simulink model "mech_bouncing_ball"  (Simulink 6.0)
settings: Solver=ode15s  StartTime=0.0  StopTime=20  FixedStep=.01  RelTol=1e-3
PreLoadFcn:
  | ball.radius = 0.2; ball.pengain = 1e5;
  | ball.mass = 1; ball.pendamp = 25;
values from neighbouring files (symbols this model uses):
  m = 161    [mech_transmission_data.mat]
  N = 270    [mech_transmission_data.mat]
libraries: mblibv1 x8
settings Model: Creator=jwendlan  LastModifiedBy=batserve  ExtModeAutoUpdateStatusClock=off  ProdHWDeviceType=Specified
settings DataIOCC: SignalLoggingName=sigsOut  OutputOption=SpecifiedOutputTimes  OutputTimes=[0:0.1:20]  Refine=3
settings DebuggingCC: CheckExecutionContextPreStartOutputMsg=on  CheckExecutionContextRuntimeOutputMsg=on  SolverPrmCheckMsg=none
settings HardwareCC: ProdHWDeviceType=Specified
settings CodeAppCC: MangleLength=5
settings SimMechanicsCC: VisOnUpdateDiagram=on  VisDuringSimulation=on  VisConfigFile=mech_bouncing_ball.mat

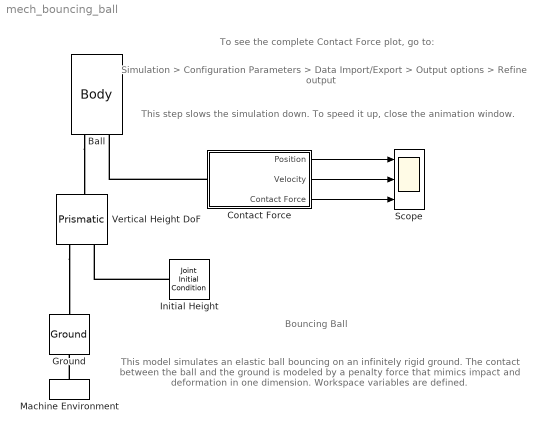
== system mech_bouncing_ball ==
  note: Bouncing Ball
  note: This model simulates an elastic ball bouncing on
      | an infinitely rigid ground. The contact between
      | the ball and the ground is modeled by a penalty force
      | that mimics impact and deformation in
      | one dimension. Workspace variables are defined.
  note: To see the complete Contact Force plot, go to:
  note: Simulation > Configuration Parameters >
      | Data Import/Export > Output options >
      | Refine output
  note: This step slows the simulation down. To speed it
      | up, close the animation window.
  Ball : mblibv1/Bodies/Body  Orientation=up  PhysicalDomain=mechanical  SubClassName=Unknown  LeftPortType=workingframe  RightPortType=workingframe  LConnTagsString=CS1|CG  DialogClass=MechanicalBodyBlock  Mass=ball.mass  MassUnits=kg  InertiaUnits=kg*m^2  Inertia=eye(3)*(2/5)*ball.mass*ball.radius^2  Shape=Cylinder  ShapeDims=[1 1]  ShapeUnits=m  ShapeUse=false  Density=1  DensityUnits=kg/m^3  DensityUse=false  CG=Left$CG$[0 0 ball.radius]$CS1$CS1$m$[0 0 0]$Euler X-Y-Z$deg$WORLD$true  WorkingFrames=Left$CS1$[0 0 0]$ADJOINING$ADJOINING$m$[0 0 0]$Euler X-Y-Z$deg$WORLD$true
  Contact Force : Subsystem
  Ground : mblibv1/Bodies/Ground  Orientation=up  Opaque=on  LeftPortType=env  RightPortType=workingframe  PhysicalDomain=Mechanical  DialogClass=GroundBlock  CoordPosition=[0 0 0]  CoordPositionUnits=m  StateVectorMgrId=-1  MachineId=[0 0]  ShowEnvPort=on
  Initial Height : mblibv1/Sensors &  Actuators/Joint Initial Condition  Orientation=left  Opaque=on  PhysicalDomain=Mechanical  DialogClass=InitialConditionBlock  InitialConditions=P1$true$5$m$rad$0$m/s$rad/s#P2$false$0$m$rad$0$m/s$rad/s#P3$false$0$m$rad$0$m/s$rad/s#R1$false$0$m$rad$0$m/s$rad/s#R2$false$0$m$rad$0$m/s$rad/s#R3$false$0$m$rad$0$m/s$rad/s#S$false$0$m$rad$0$m/s$rad/s
  Machine Environment : mblibv1/Bodies/Machine Environment  Tag=Factory ground  Orientation=up  DialogController=MECH.DialogSource  Opaque=on  PortType=env  PhysicalDomain=Mechanical  DialogTemplateClass=MECH.MachineEnvironment  SyncWhenCopied=off  Gravity=[0 0 -9.81]  GravityUnits=m/s^2  GravityAsSignal=off  Dimensionality=3D Only  AnalysisType=Forward dynamics  LinearAssemblyTolerance=1e-3  LinearAssemblyToleranceUnits=m  AngularAssemblyTolerance=1e-3  AngularAssemblyToleranceUnits=rad  ConstraintSolverType=Stabilizing  ConstraintRelTolerance=1e-4  ConstraintAbsTolerance=1e-4  UseRobustSingularityHandling=off  StatePerturbationType=Fixed  PerturbationSize=1e-5  VisualizeMachine=on
  Scope : Scope  NumInputPorts=3
      settings: TimeRange=20  YMin=0~-10~0  YMax=6~10~3000  MaxDataPoints=50000
  Vertical Height DoF : mblibv1/Joints/Prismatic  Orientation=up  PhysicalDomain=mechanical  SubClassName=Unknown  LeftPortType=blob  RightPortType=blob  LConnTagsString=__newl0|SA1  RConnTagsString=__newr0  NumSAPorts=1  CutJoint=off  MarkAsCut=off  Primitives=prismatic  PrimitiveProps=P1$WORLD$[0 0 1]$prismatic  DialogClass=JointBlock
  wires:
  Contact Force/1(Position) -> Scope/1
  Contact Force/2(Velocity) -> Scope/2
  Contact Force/3(Contact Force) -> Scope/3
  connections:
  Vertical Height DoF/LConn1 -- Ground/RConn1
  Initial Height/RConn1 -- Vertical Height DoF/LConn2
  Ball/LConn1 -- Vertical Height DoF/RConn1
  Contact Force/LConn1 -- Ball/LConn2
  Machine Environment/RConn1 -- Ground/LConn1

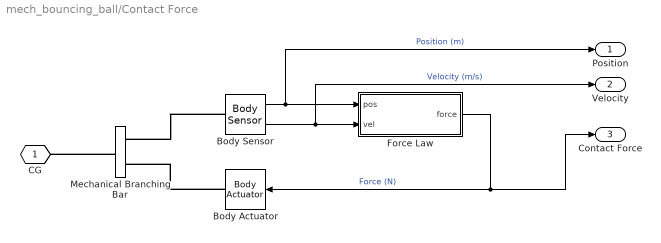
== system mech_bouncing_ball/Contact Force ==
  Body Actuator : mblibv1/Sensors &  Actuators/Body Actuator  Orientation=left  Opaque=on  PhysicalDomain=Mechanical  PortType=blob  ActuationStyle=Force  AngleUnits=deg  ArcVelocityUnits=deg/s  ArcAccelerationUnits=deg/s^2  CoordPositionUnits=m  VelocityUnits=m/s  AccelerationUnits=m/s^2  ForceUnits=N  TorqueUnits=N-m  ActiveIO=on  Width=3  DialogClass=MechanicalActuatorBlock  ReferenceFrame=Absolute (INERTIAL)  Angle=off  CoordPosition=on  Force=on  Torque=off
  Body Sensor : mblibv1/Sensors &  Actuators/Body Sensor  Opaque=on  PhysicalDomain=Mechanical  PortType=blob  Muxed=off  Pose=off  Angle=on  AngleUnits=deg  ArcVelocity=off  ArcVelocityUnits=deg/s  ArcAcceleration=off  ArcAccelerationUnits=deg/s^2  CoordPosition=on  CoordPositionUnits=m  Velocity=on  VelocityUnits=m/s  Acceleration=off  AccelerationUnits=m/s^2  Quaternion=on  QuaternionDT=off  QuaternionDDT=off  QuaternionUnits=off  OutputVector=[ 3 3 ]  ActiveIO=on  Width=6  DialogClass=MechanicalSensorBlock  ReferenceFrame=Absolute (World)
  Force Law : Subsystem
  Mechanical Branching Bar : mblibv1/Utilities/Mechanical Branching Bar  PhysicalDomain=mechanical  SubClassName=Unknown  LeftPortType=blob  RightPortType=blob  LConnTagsString=_newl0  RConnTagsString=SA0|SA1  DialogClass=MechanicalBranchingBarBlock  NumSAPorts=2
  CG : PMIOPort  Tag=PMCPort  Port=1  Side=Left
  Position : Outport
  Velocity : Outport  Port=2
  Contact Force : Outport  Port=3
  wires:
  Body Sensor/1 -> Force Law/1(pos), Position/1  "Position (m)"
  Body Sensor/2 -> Force Law/2(vel), Velocity/1  "Velocity (m/s)"
  Force Law/1(force) -> Body Actuator/1, Contact Force/1  "Force (N)"
  connections:
  Mechanical Branching Bar/LConn1 -- CG/RConn1
  Body Actuator/RConn1 -- Mechanical Branching Bar/RConn2
  Body Sensor/LConn1 -- Mechanical Branching Bar/RConn1

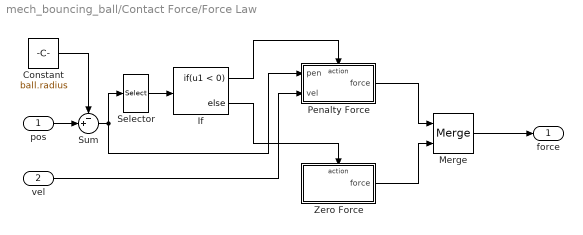
== system mech_bouncing_ball/Contact Force/Force Law ==
  pos : Inport  Port=1  LatchInput=off
  vel : Inport  Port=2  LatchInput=off
  Constant : Constant  Value=ball.radius
  If : If  IfExpression=u1 < 0
  Merge : Merge  InitialOutput=0  InputPortOffsets=0
  Penalty Force : Subsystem  TreatAsAtomicUnit=on
  Selector : Selector  Elements=[3]  InputPortWidth=3
  Sum : Sum  Inputs=-+|  SaturateOnIntegerOverflow=on
  Zero Force : Subsystem  TreatAsAtomicUnit=on
  force : Outport
  wires:
  pos/1 -> Sum/2
  Sum/1 -> Selector/1, Penalty Force/1(pen)
  Constant/1 -> Sum/1
  vel/1 -> Penalty Force/2(vel)
  If/2 -> Zero Force/Action
  Penalty Force/1(force) -> Merge/1
  Zero Force/1(force) -> Merge/2
  Merge/1 -> force/1
  If/1 -> Penalty Force/Action
  Selector/1 -> If/1

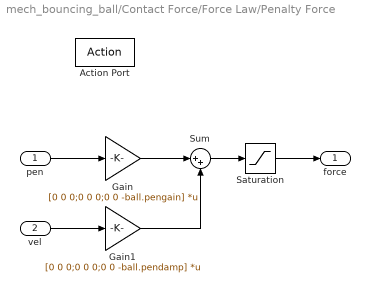
== system mech_bouncing_ball/Contact Force/Force Law/Penalty Force ==
  pen : Inport  Port=1  LatchInput=off
  vel : Inport  Port=2  LatchInput=off
  Action Port : ActionPort  ActionType=then
  Gain : Gain  Gain=[0 0 0;0 0 0;0 0 -ball.pengain]  Multiplication=Matrix(K*u)  SaturateOnIntegerOverflow=on
  Gain1 : Gain  Gain=[0 0 0;0 0 0;0 0 -ball.pendamp]  Multiplication=Matrix(K*u)  SaturateOnIntegerOverflow=on
  Saturation : Saturate  UpperLimit=inf  LowerLimit=0
  Sum : Sum  Inputs=|++  SaturateOnIntegerOverflow=on
  force : Outport  InitialOutput=0
  wires:
  pen/1 -> Gain/1
  Gain/1 -> Sum/1
  Sum/1 -> Saturation/1
  Gain1/1 -> Sum/2
  vel/1 -> Gain1/1
  Saturation/1 -> force/1

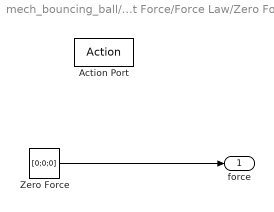
== system mech_bouncing_ball/Contact Force/Force Law/Zero Force ==
  Action Port : ActionPort  ActionType=else
  Zero Force : Constant  Value=[0;0;0]
  force : Outport  InitialOutput=0
  wires:
  Zero Force/1 -> force/1
